simulink model "Quanser_Experimental"  (R2017b)
settings: Solver=ode1  StartTime=0.0  StopTime=inf  FixedStep=0.002  RelTol=1e-3  EnableMultiTasking=on
values from neighbouring files (symbols this model uses):
  A = [0,1,0,0,0,0;0,0,0,0,0,0;0,0,0,1,0,0;0,0,0,0,0,0;0,0,0,0,0,1;0,0,0,0,0,0]    [ProportionalController.m]    (also in SecondOrderResponse.m = (log(PO/100))^2)
  B = [0,0,0;(1/Ix),0,0;0,0,0;0,(1/Iy),0;0,0,0;0,0,(1/Iz)]    [ProportionalController.m]
  C = [1,0,0,0,0,0;0,1,0,0,0,0;0,0,1,0,0,0]    [ProportionalController.m]
  CMD_RATE_LIMIT = 60 * pi/180    (= 1.0471975512)    [ProportionalController.m]
  D = [0,0,0;0,0,0;0,0,0]    [ProportionalController.m]
  K_AMP = 3    [ProportionalController.m]
  V_bias = 2    [ProportionalController.m]
  VMAX_AMP = 24    [ProportionalController.m]
  wcf = 2 * pi * 20    (= 125.663706144)    [ProportionalController.m]
  zetaf = 0.6    [ProportionalController.m]
undefined symbols (not defined in the file or in its folder): Continuous, HIL, INT_JOYSTICK_SAT_LOWER, INT_JOYSTICK_SAT_UPPER, JOYSTICK_X_DZ, JOYSTICK_Y_DZ, K_EC_P, K_EC_R, K_EC_Y, K_JOYSTICK_X, K_JOYSTICK_Y, KiLQRI, KmLQRI, KmLQRI_prime, qc_get_step_size, Time
libraries: simulink_extras x9, quarc_library x4, simulink x3, ctrlSharedLib x1
settings Model: SimulationMode=external  ExtModeTrigDuration=10000  Creator=hpineros  LastModifiedBy=YvesDaoud
settings SolverCC: PositivePriorityOrder=on
settings DataIOCC: LimitDataPoints=on  SaveFormat=Array  SignalLoggingSaveFormat=ModelDataLogs
settings OptimizationCC: ExpressionDepthLimit=2147483647  InitFltsAndDblsToZero=on  LifeSpan=inf
settings DebuggingCC: SaveWithParameterizedLinksMsg=none  UnderspecifiedInitializationDetection=Classic  MergeDetectMultiDrivingBlocksExec=none  SolverPrmCheckMsg=warning  FcnCallInpInsideContextMsg=warning  AllowSymbolicDim=off  StateNameClashWarn=warning  SFUnexpectedBacktrackingDiag=warning  SFNoUnconditionalDefaultTransitionDiag=warning  SFExecutionAtInitializationDiag=none
settings HardwareCC: ProdBitPerPointer=32  ProdBitPerSizeT=32  ProdBitPerPtrDiffT=32  ProdLargestAtomicFloat=None  ProdIntDivRoundTo=Undefined  ProdEndianess=Unspecified  ProdWordSize=32  ProdHWDeviceType=32-bit Generic
settings ModelReferenceCC: PropagateSignalLabelsOutOfModel=off
settings RTWCC: SystemTargetFile=quarc_win64.tlc  TemplateMakefile=quarc_default_tmf  Description=QUARC Win64 Target
settings CodeAppCC: StateflowObjectComments=on
settings STFCustomTargetCC: TargetPreCompLibLocation=C:\PROGRA~3\QUARC\lib\2015b\win64\release  ConcurrentExecutionCompliant=on  GeneratePreprocessorConditionals=Disable all  CombineOutputUpdateFcns=on  CPPClassGenCompliant=on  GRTInterface=off  SystemTargetFile=quarc_win64.tlc
settings GRTTargetCC: TargetPreCompLibLocation=C:\PROGRA~3\QUARC\lib\2015b\win64\release  TargetLangStandard=C89/C90 (ANSI)  ParMdlRefBuildCompliant=off  CompOptLevelCompliant=off  GeneratePreprocessorConditionals=Disable all  MatFileLogging=off  UseToolchainInfoCompliant=off  ExtMode=on  ExtModeMexFile=quarc_comm
settings ConfigComp: CovMetricSettings=dw  CovHtmlReporting=on  CovSaveCumulativeToWorkspaceVar=on  CovSaveSingleToWorkspaceVar=on  CovExternalEMLEnable=off

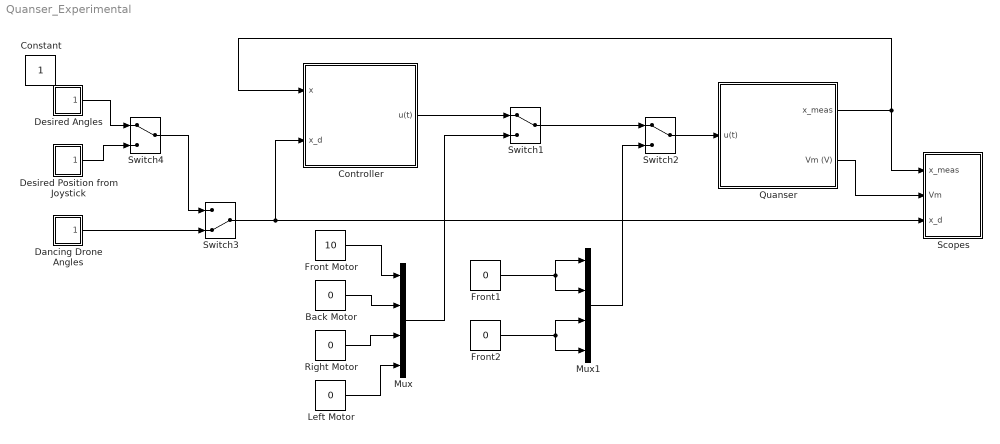
== system Quanser_Experimental ==
  Back Motor : Constant  Value=0
  Controller : Subsystem
  Dancing Drone Angles : Subsystem
  Desired Angles : Subsystem
  Desired Position from Joystick : Subsystem
  Front Motor : Constant  Value=10
  Front1 : Constant  Value=0
  Front2 : Constant  Value=0
  Left Motor : Constant  Value=0
  Mux : Mux
  Mux1 : Mux
  Quanser : Subsystem
  Right Motor : Constant  Value=0
  Scopes : Subsystem
  Switch1 : ManualSwitch
  Switch2 : ManualSwitch
  Switch3 : ManualSwitch  CurrentSetting=0
  Switch4 : ManualSwitch
  Constant : Constant  IOType=siggen
  wires:
  Quanser/1(x_meas) -> Controller/1(x), Scopes/1(x_meas)
  Quanser/2(Vm (V)) -> Scopes/2(Vm)
  Desired Angles/1(x_d) -> Switch4/1
  Desired Position from Joystick/1(x_d) -> Switch4/2
  Controller/1(u(t)) -> Switch1/1
  Mux/1 -> Switch1/2
  Front Motor/1 -> Mux/1
  Back Motor/1 -> Mux/2
  Right Motor/1 -> Mux/3
  Left Motor/1 -> Mux/4
  Mux1/1 -> Switch2/2
  Front1/1 -> Mux1/1, Mux1/2
  Switch1/1 -> Switch2/1
  Switch2/1 -> Quanser/1(u(t))
  Front2/1 -> Mux1/4, Mux1/3
  Switch3/1 -> Controller/2(x_d), Scopes/3(x_d)
  Switch4/1 -> Switch3/1
  Dancing Drone Angles/1(x_d) -> Switch3/2

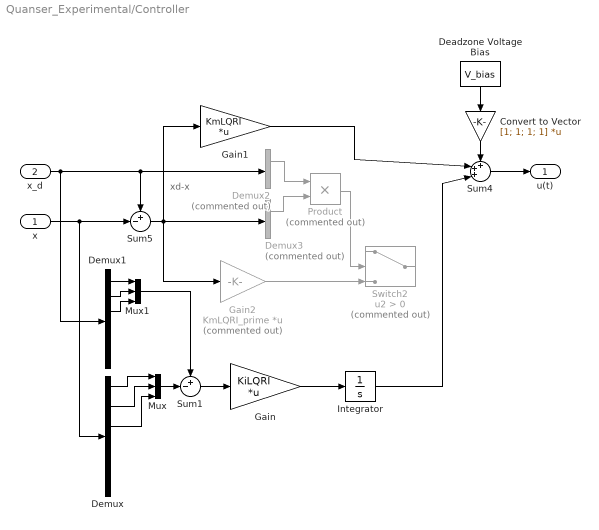
== system Quanser_Experimental/Controller ==
  note: xd-x
  x : Inport
  x_d : Inport  Port=2
  Convert to Vector : Gain  Gain=[1; 1; 1; 1]  Multiplication=Matrix(K*u)
  Deadzone Voltage Bias : Constant  Value=V_bias
  Demux : Demux  Outputs=6
  Demux1 : Demux  Outputs=6
  Demux2 : Demux  Commented=on  Outputs=6
  Demux3 : Demux  Commented=on  Outputs=6
  Gain : Gain  Gain=KiLQRI  Multiplication=Matrix(K*u)
  Gain1 : Gain  Gain=KmLQRI  Multiplication=Matrix(K*u)
  Gain2 : Gain  Commented=on  Gain=KmLQRI_prime  Multiplication=Matrix(K*u)
  Integrator : Integrator
  Mux : Mux  Inputs=3
  Mux1 : Mux  Inputs=3
  Product : Product  Commented=on
  Sum1 : Sum  Inputs=+-|
  Sum4 : Sum  Inputs=+++|
  Sum5 : Sum  Inputs=+-|
  Switch2 : Switch  Commented=on  Criteria=u2 > Threshold
  u(t) : Outport
  wires:
  Sum5/1 -> Gain1/1, Demux3/1, Gain2/1
  x/1 -> Demux/1, Sum5/2
  Convert to Vector/1 -> Sum4/1
  Deadzone Voltage Bias/1 -> Convert to Vector/1
  Sum4/1 -> u(t)/1
  Demux/1 -> Mux/1
  Demux/2 -> Mux/2
  Demux/3 -> Mux/3
  Mux/1 -> Sum1/2
  Gain/1 -> Integrator/1
  Sum1/1 -> Gain/1
  Integrator/1 -> Sum4/3
  x_d/1 -> Demux2/1, Sum5/1, Demux1/1
  Demux1/1 -> Mux1/1
  Demux1/2 -> Mux1/2
  Demux1/3 -> Mux1/3
  Mux1/1 -> Sum1/1
  Gain1/1 -> Sum4/2
  Gain2/1 -> Switch2/3
  Product/1 -> Switch2/2
  Demux2/2 -> Product/1
  Demux3/2 -> Product/2

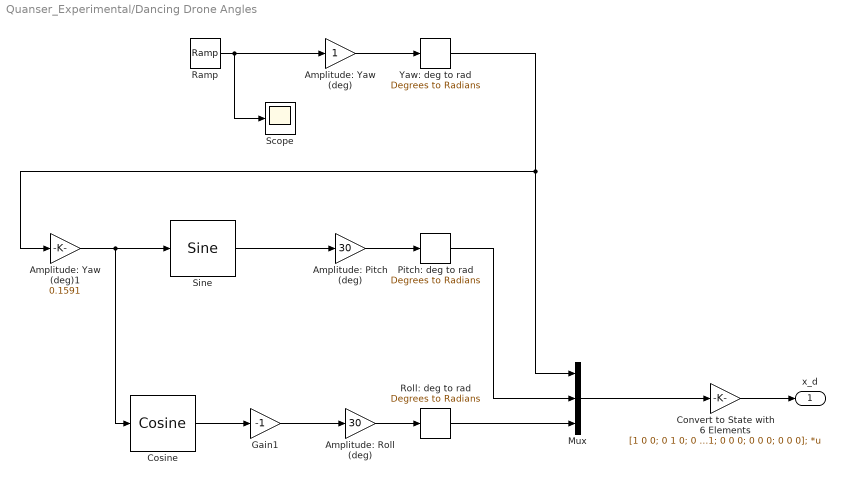
== system Quanser_Experimental/Dancing Drone Angles ==
  Amplitude: Pitch (deg) : Gain  Gain=30
  Amplitude: Roll (deg) : Gain  Gain=30
  Amplitude: Yaw (deg) : Gain
  Amplitude: Yaw (deg)1 : Gain  Gain=0.1591
  Convert to State with 6 Elements : Gain  Gain=[1 0 0; 0 1 0; 0 0 1; 0 0 0; 0 0 0; 0 0 0];  Multiplication=Matrix(K*u)
  Cosine : simulink/Lookup Tables/Cosine  Formula=cos(2*pi*u)  NumDataPoints=(2^5)+1  OutputWordLength=16  InternalRulePriority=Speed
      settings: SourceProductName=Simulink  SourceProductBaseCode=SL
  Gain1 : Gain  Gain=-1
  Mux : Mux  Inputs=3
  Pitch: deg to rad : simulink_extras/Transformations/Degrees to Radians
  Ramp : simulink/Sources/Ramp  slope=-20  start=0  X0=0
  Roll: deg to rad : simulink_extras/Transformations/Degrees to Radians
  Scope : Scope
  Sine : simulink/Lookup Tables/Sine  Formula=sin(2*pi*u)  NumDataPoints=(2^5)+1  OutputWordLength=16  InternalRulePriority=Speed
      settings: SourceProductName=Simulink
  Yaw: deg to rad : simulink_extras/Transformations/Degrees to Radians
  x_d : Outport
  wires:
  Convert to State with 6 Elements/1 -> x_d/1
  Mux/1 -> Convert to State with 6 Elements/1
  Roll: deg to rad/1 -> Mux/3
  Pitch: deg to rad/1 -> Mux/2
  Amplitude: Roll (deg)/1 -> Roll: deg to rad/1
  Amplitude: Pitch (deg)/1 -> Pitch: deg to rad/1
  Amplitude: Yaw (deg)/1 -> Yaw: deg to rad/1
  Sine/1 -> Amplitude: Pitch (deg)/1
  Yaw: deg to rad/1 -> Mux/1, Amplitude: Yaw (deg)1/1
  Cosine/1 -> Gain1/1
  Gain1/1 -> Amplitude: Roll (deg)/1
  Amplitude: Yaw (deg)1/1 -> Cosine/1, Sine/1
  Ramp/1 -> Scope/1, Amplitude: Yaw (deg)/1

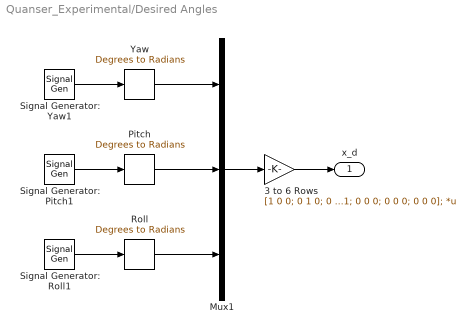
== system Quanser_Experimental/Desired Angles ==
  3 to 6 Rows : Gain  Gain=[1 0 0; 0 1 0; 0 0 1; 0 0 0; 0 0 0; 0 0 0];  Multiplication=Matrix(K*u)
  Mux1 : Mux  Inputs=3
  Pitch : simulink_extras/Transformations/Degrees to Radians
  Roll : simulink_extras/Transformations/Degrees to Radians
  Signal Generator: Pitch1 : SignalGenerator  WaveForm=square  Amplitude=5  Frequency=0.04
  Signal Generator: Roll1 : SignalGenerator  WaveForm=square  Amplitude=5  Frequency=0.04
  Signal Generator: Yaw1 : SignalGenerator  WaveForm=square  Amplitude=5  Frequency=0.04
  Yaw : simulink_extras/Transformations/Degrees to Radians
  x_d : Outport
  wires:
  3 to 6 Rows/1 -> x_d/1
  Signal Generator: Yaw1/1 -> Yaw/1
  Signal Generator: Pitch1/1 -> Pitch/1
  Signal Generator: Roll1/1 -> Roll/1
  Yaw/1 -> Mux1/1
  Pitch/1 -> Mux1/2
  Roll/1 -> Mux1/3
  Mux1/1 -> 3 to 6 Rows/1

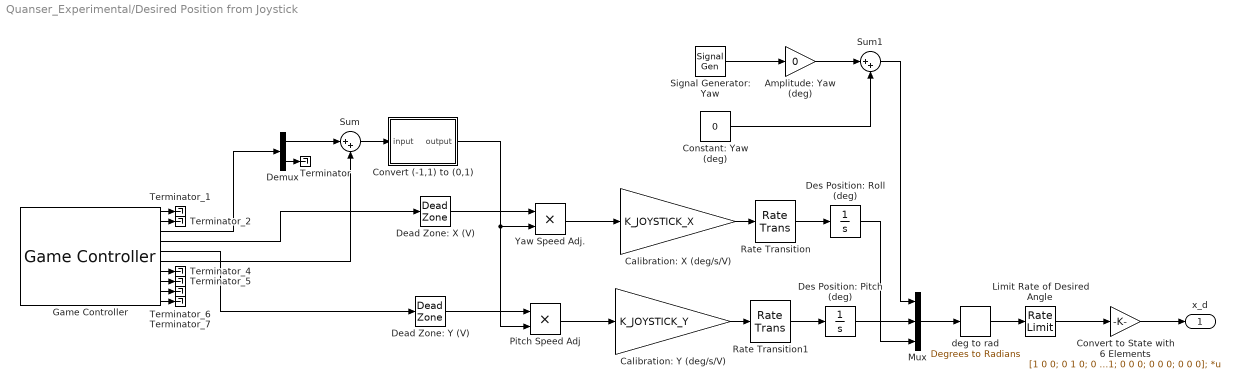
== system Quanser_Experimental/Desired Position from Joystick ==
  Amplitude: Yaw (deg) : Gain  Gain=0
  Calibration: X (deg/s/V) : Gain  Gain=K_JOYSTICK_X
  Calibration: Y (deg/s/V) : Gain  Gain=K_JOYSTICK_Y
  Constant: Yaw (deg) : Constant  Value=0
  Convert (-1,1) to (0,1) : Subsystem
  Convert to State with 6 Elements : Gain  Gain=[1 0 0; 0 1 0; 0 0 1; 0 0 0; 0 0 0; 0 0 0];  Multiplication=Matrix(K*u)
  Dead Zone: X (V) : DeadZone  LowerValue=-JOYSTICK_X_DZ  UpperValue=JOYSTICK_X_DZ  SaturateOnIntegerOverflow=on
  Dead Zone: Y (V) : DeadZone  LowerValue=-JOYSTICK_Y_DZ  UpperValue=JOYSTICK_Y_DZ  SaturateOnIntegerOverflow=on
  Demux : Demux  Outputs=2
  Des Position: Pitch (deg) : Integrator  LimitOutput=on  UpperSaturationLimit=INT_JOYSTICK_SAT_UPPER  LowerSaturationLimit=INT_JOYSTICK_SAT_LOWER
  Des Position: Roll (deg) : Integrator  LimitOutput=on  UpperSaturationLimit=INT_JOYSTICK_SAT_UPPER  LowerSaturationLimit=INT_JOYSTICK_SAT_LOWER
  Game Controller : quarc_library/Devices/Peripherals/Target/Game Controller  controller=1  buffer_size=12  deadzone=[]  saturation=[]  sample_time=max(qc_get_step_size, 0.01)  auto_center=off  enabled=on
  Limit Rate of Desired Angle : RateLimiter  RisingSlewLimit=CMD_RATE_LIMIT  FallingSlewLimit=-CMD_RATE_LIMIT
  Mux : Mux  Inputs=3
  Pitch Speed Adj : Product  RndMeth=Zero
  Rate Transition : RateTransition
  Rate Transition1 : RateTransition
  Signal Generator: Yaw : SignalGenerator  WaveForm=square  Frequency=0.04
  Sum : Sum  Inputs=|++
  Sum1 : Sum  Inputs=|++
  Terminator : Terminator
  Terminator_{1..2,4..7} (6 alike) : Terminator
  Yaw Speed Adj. : Product  RndMeth=Zero
  deg to rad : simulink_extras/Transformations/Degrees to Radians
  x_d : Outport
  wires:
  Sum1/1 -> Mux/1
  Signal Generator: Yaw/1 -> Amplitude: Yaw (deg)/1
  Amplitude: Yaw (deg)/1 -> Sum1/1
  Constant: Yaw (deg)/1 -> Sum1/2
  Limit Rate of Desired Angle/1 -> Convert to State with 6 Elements/1
  Mux/1 -> deg to rad/1
  deg to rad/1 -> Limit Rate of Desired Angle/1
  Convert to State with 6 Elements/1 -> x_d/1
  Calibration: X (deg/s/V)/1 -> Rate Transition/1
  Dead Zone: X (V)/1 -> Yaw Speed Adj./1
  Dead Zone: Y (V)/1 -> Pitch Speed Adj/1
  Yaw Speed Adj./1 -> Calibration: X (deg/s/V)/1
  Pitch Speed Adj/1 -> Calibration: Y (deg/s/V)/1
  Calibration: Y (deg/s/V)/1 -> Rate Transition1/1
  Convert (-1,1) to (0,1)/1(output) -> Yaw Speed Adj./2, Pitch Speed Adj/2
  Rate Transition/1 -> Des Position: Roll (deg)/1
  Des Position: Roll (deg)/1 -> Mux/3
  Des Position: Pitch (deg)/1 -> Mux/2
  Rate Transition1/1 -> Des Position: Pitch (deg)/1
  Game Controller/4 -> Dead Zone: X (V)/1
  Game Controller/5 -> Dead Zone: Y (V)/1
  Game Controller/1 -> Terminator_1/1
  Game Controller/2 -> Terminator_2/1
  Game Controller/7 -> Terminator_4/1
  Game Controller/8 -> Terminator_5/1
  Game Controller/9 -> Terminator_6/1
  Game Controller/10 -> Terminator_7/1
  Sum/1 -> Convert (-1,1) to (0,1)/1(input)
  Game Controller/6 -> Sum/2
  Demux/1 -> Sum/1
  Game Controller/3 -> Demux/1
  Demux/2 -> Terminator/1

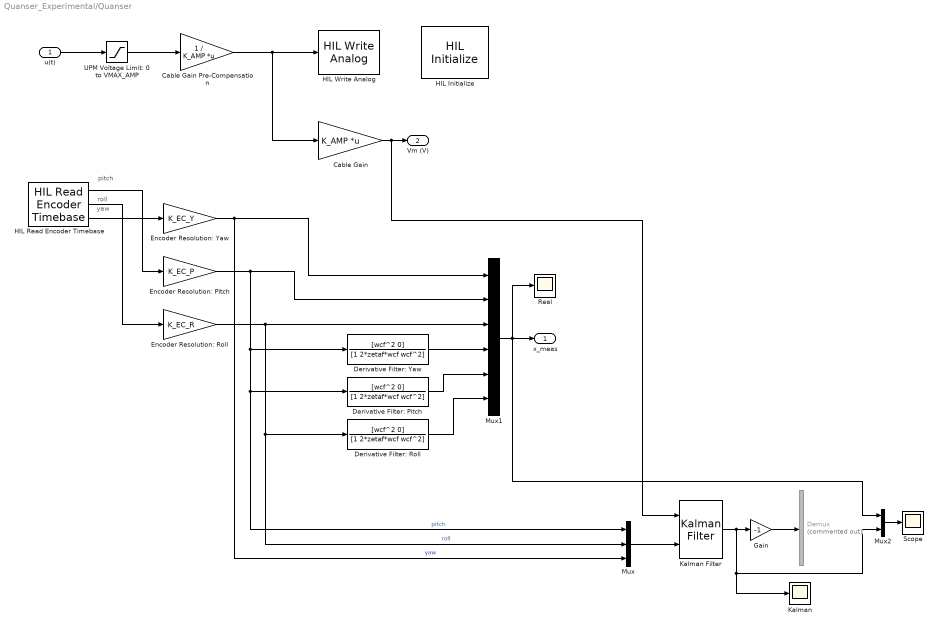
== system Quanser_Experimental/Quanser ==
  note: roll
  note: pitch
  note: yaw
  u(t) : Inport
  Cable Gain : Gain  Gain=K_AMP  Multiplication=Matrix(K*u)  SaturateOnIntegerOverflow=on  OutDataTypeStr=Inherit: Same as input  ParamDataTypeStr=Inherit: Same as input
  Cable Gain Pre-Compensation : Gain  Gain=1 / K_AMP  Multiplication=Matrix(K*u)  SaturateOnIntegerOverflow=on  OutDataTypeStr=Inherit: Same as input  ParamDataTypeStr=Inherit: Same as input
  Demux : Demux  Commented=on  Outputs=6
  Derivative Filter: Pitch : TransferFcn  Numerator=[wcf^2 0]  Denominator=[1 2*zetaf*wcf wcf^2]
  Derivative Filter: Roll : TransferFcn  Numerator=[wcf^2 0]  Denominator=[1 2*zetaf*wcf wcf^2]
  Derivative Filter: Yaw : TransferFcn  Numerator=[wcf^2 0]  Denominator=[1 2*zetaf*wcf wcf^2]
  Encoder Resolution: Pitch : Gain  Gain=K_EC_P
  "Encoder Resolution: Roll " : Gain  Gain=K_EC_R
  Encoder Resolution: Yaw : Gain  Gain=K_EC_Y
  Gain : Gain  Gain=-1
  HIL Initialize : quarc_library/Data Acquisition/Generic/Configuration/HIL Initialize  object_name=HIL-1  board_type=q8_usb  board_number=0  board_options=update_rate=normal;decimation=1  exclusive=off  active=on  hardware_clocks=[0:2]  clock_modes=[]  initial_clock_frequencies=[]  set_clock_params_at_start=off  set_clock_params_at_switch_in=off  set_clock_frequencies_at_start=off  set_clock_frequencies_at_switch_in=off  analog_input_channels=[0:7]  analog_input_maximums=10  analog_input_minimums=-10  set_analog_input_params_at_start=on  set_analog_input_params_at_switch_in=off  analog_output_channels=[0:7]  analog_output_maximums=10  analog_output_minimums=-10  initial_analog_outputs=[0]  final_analog_outputs=[0]  watchdog_analog_outputs=0  set_analog_output_params_at_start=on  set_analog_output_params_at_switch_in=off  set_analog_outputs_at_start=on  set_analog_outputs_at_switch_in=off  set_analog_outputs_at_terminate=on  set_analog_outputs_at_switch_out=off  set_analog_outputs_on_watchdog=off  digital_input_channels=[]  digital_output_channels=[]  digital_output_configuration=[]  initial_digital_outputs=[1]  final_digital_outputs=[1]  watchdog_digital_outputs=[1]  set_digital_output_params_at_start=off  set_digital_output_params_at_switch_in=off  set_digital_outputs_at_start=on  set_digital_outputs_at_switch_in=off  set_digital_outputs_at_terminate=on  set_digital_outputs_at_switch_out=off  set_digital_outputs_on_watchdog=off  encoder_channels=[0:7]  quadrature=[4]  encoder_filter_frequency=[]  initial_encoder_counts=[0]  set_encoder_params_at_start=on  set_encoder_params_at_switch_in=off  set_encoder_counts_at_start=on  set_encoder_counts_at_switch_in=off  pwm_channels=[0:7]  pwm_modes=0  pwm_frequency=99.532799999999995e6/4095  pwm_configuration=[0]  pwm_alignment=[0]  pwm_polarity=[1]  pwm_leading_deadband=[0]  pwm_trailing_deadband=[0]  initial_pwm_outputs=[0]  final_pwm_outputs=[0]  watchdog_pwm_outputs=[0]  set_pwm_params_at_start=on  set_pwm_params_at_switch_in=off  set_pwm_outputs_at_start=on  set_pwm_outputs_at_switch_in=off  set_pwm_outputs_at_terminate=on  set_pwm_outputs_at_switch_out=off  set_pwm_outputs_on_watchdog=off  other_output_channels=[]  initial_other_outputs=[]  final_other_outputs=[]  watchdog_other_outputs=[]  set_other_outputs_at_start=off  set_other_outputs_at_switch_in=off  set_other_outputs_at_terminate=off  set_other_outputs_at_switch_out=off  set_other_outputs_on_watchdog=off
  HIL Read Encoder Timebase : quarc_library/Data Acquisition/Generic/Timebases/HIL Read Encoder Timebase  object_name=HIL-1  clock=0  channels=[0:2]  samples_in_buffer=max(ceil(1/qc_get_step_size), 1)  active=on  vector_output=off  data_type_mode=Inherit via back propagation  data_type=double
  HIL Write Analog : quarc_library/Data Acquisition/Generic/Immediate I//O/HIL Write Analog  object_name=HIL-1  channels=[0,1,3,2]  sample_time=-1  active=off  vector_input=on
  Kalman : Scope
  Kalman Filter : ctrlSharedLib/Kalman Filter  TimeDomain=Continuous-Time  UseCurrentEstimator=on  ModelSource=Individual A, B, C, D matrices  ModelSourceVariable=ss(0.95,1,1,0,1)  A=A  B=B  C=C  D=D  NumberOfStates=1  NumberOfInputs=1  NumberOfOutputs=1  InitialEstimateSource=Dialog  X0=0  P0=10  UseK=off  UseGH=off  NumberOfProcessNoiseInputs=1  G=1  TimeInvariantG=on  H=0  TimeInvariantH=on  Q=0.05  TimeInvariantQ=on  R=1  TimeInvariantR=on  N=0  TimeInvariantN=on  AddInputPort=on  AddEnablePort=off  OutputEstimatedY=off  OutputP=off  Ts=-1
      settings: SourceProductBaseCode=CT
  Mux : Mux  Inputs=3
  Mux1 : Mux  Inputs=6
  Mux2 : Mux  Inputs=2
  Real : Scope
  Scope : Scope
  UPM Voltage Limit: 0 to VMAX_AMP : Saturate  UpperLimit=VMAX_AMP  LowerLimit=1
  x_meas : Outport
  Vm (V) : Outport  Port=2
  wires:
  Cable Gain Pre-Compensation/1 -> Cable Gain/1, HIL Write Analog/1
  HIL Read Encoder Timebase/3 -> Encoder Resolution: Yaw/1
  HIL Read Encoder Timebase/1 -> Encoder Resolution: Pitch/1
  HIL Read Encoder Timebase/2 -> "Encoder Resolution: Roll "/1
  UPM Voltage Limit: 0 to VMAX_AMP/1 -> Cable Gain Pre-Compensation/1
  Cable Gain/1 -> Kalman Filter/1, Vm (V)/1
  u(t)/1 -> UPM Voltage Limit: 0 to VMAX_AMP/1
  Encoder Resolution: Yaw/1 -> Mux1/1, Mux/3  "yaw"
  Encoder Resolution: Pitch/1 -> Mux1/2, Derivative Filter: Yaw/1, Derivative Filter: Pitch/1, Mux/1  "pitch"
  "Encoder Resolution: Roll "/1 -> Mux/2, Derivative Filter: Roll/1, Mux1/3  "roll"
  Derivative Filter: Yaw/1 -> Mux1/4
  Derivative Filter: Pitch/1 -> Mux1/5
  Derivative Filter: Roll/1 -> Mux1/6
  Mux/1 -> Kalman Filter/2
  Mux2/1 -> Scope/1
  Kalman Filter/1 -> Kalman/1, Mux2/2, Gain/1
  Gain/1 -> Demux/1
  Mux1/1 -> x_meas/1, Real/1, Mux2/1

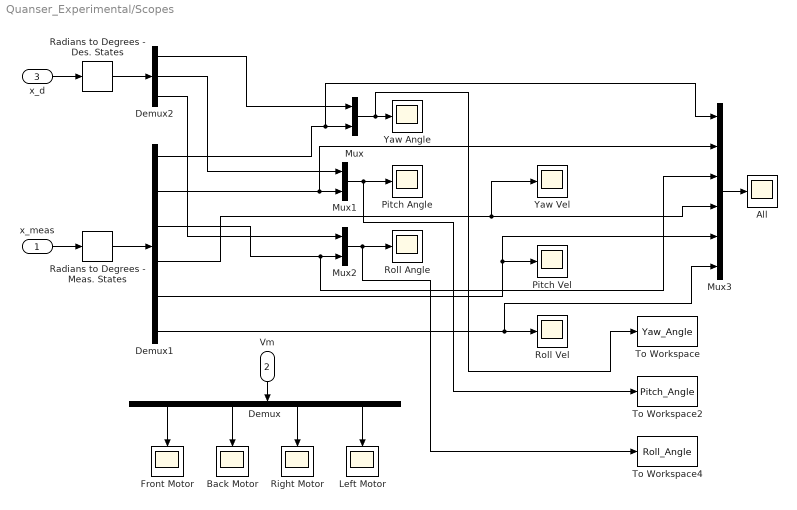
== system Quanser_Experimental/Scopes ==
  x_meas : Inport
  Vm : Inport  Port=2
  x_d : Inport  Port=3
  All : Scope
  Back Motor : Scope
  Demux : Demux
  Demux1 : Demux  Outputs=6
  Demux2 : Demux  Outputs=3
  Front Motor : Scope
  Left Motor : Scope
  Mux : Mux  Inputs=2
  Mux1 : Mux  Inputs=2
  Mux2 : Mux  Inputs=2
  Mux3 : Mux  Inputs=6
  Pitch Angle : Scope
  Pitch Vel : Scope
  Radians to Degrees - Des. States : simulink_extras/Transformations/Radians to Degrees
  Radians to Degrees - Meas. States : simulink_extras/Transformations/Radians to Degrees
  Right Motor : Scope
  Roll Angle : Scope
  Roll Vel : Scope
  To Workspace : ToWorkspace  VariableName=Yaw_Angle  SampleTime=-1
      settings: Save2DSignal=2-D array (concatenate along first dimension)
  To Workspace2 : ToWorkspace  VariableName=Pitch_Angle  SampleTime=-1
      settings: Save2DSignal=2-D array (concatenate along first dimension)
  To Workspace4 : ToWorkspace  VariableName=Roll_Angle  SampleTime=-1
      settings: Save2DSignal=2-D array (concatenate along first dimension)
  Yaw Angle : Scope
  Yaw Vel : Scope
  wires:
  Demux/4 -> Left Motor/1
  Demux/3 -> Right Motor/1
  Demux/2 -> Back Motor/1
  Demux/1 -> Front Motor/1
  Vm/1 -> Demux/1
  x_d/1 -> Radians to Degrees - Des. States/1
  x_meas/1 -> Radians to Degrees - Meas. States/1
  Mux/1 -> To Workspace/1, Yaw Angle/1
  Mux1/1 -> To Workspace2/1, Pitch Angle/1
  Mux2/1 -> To Workspace4/1, Roll Angle/1
  Radians to Degrees - Meas. States/1 -> Demux1/1
  Demux1/1 -> Mux3/1, Mux/2
  Demux1/2 -> Mux3/2, Mux1/2
  Demux1/3 -> Mux3/3, Mux2/2
  Demux1/4 -> Yaw Vel/1, Mux3/4
  Demux1/6 -> Mux3/6, Roll Vel/1
  Mux3/1 -> All/1
  Demux1/5 -> Mux3/5, Pitch Vel/1
  Radians to Degrees - Des. States/1 -> Demux2/1
  Demux2/1 -> Mux/1
  Demux2/2 -> Mux1/1
  Demux2/3 -> Mux2/1

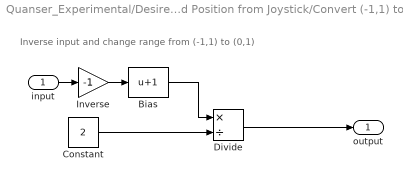
== system Quanser_Experimental/Desired Position from Joystick/Convert (-1,1) to (0,1) ==
  note: Inverse input and change range from (-1,1) to (0,1)
  input : Inport
  Bias : Bias  Bias=1
  Constant : Constant  Value=2
  Divide : Product  Inputs=*/
  Inverse : Gain  Gain=-1
  output : Outport
  wires:
  Bias/1 -> Divide/1
  input/1 -> Inverse/1
  Divide/1 -> output/1
  Inverse/1 -> Bias/1
  Constant/1 -> Divide/2
